simulink model "block_diagram_for_three_phase_vsi"  (R2014a)
settings: Solver=ode23t  StartTime=0.0  StopTime=1  MaxStep=1e-6  RelTol=1e-3
values from neighbouring files (symbols this model uses):
  p11 = rem(m,360)    [code_for_single_phase_csi.m]    (also in code_for_single_phase_vsi.m; code_for_three_phase_csi.m; code_for_three_phase_vsi.m; code_for_vsi.m)
  p22 = rem(n,360)    [code_for_single_phase_csi.m]    (also in code_for_single_phase_vsi.m; code_for_three_phase_csi.m; code_for_three_phase_vsi.m; code_for_vsi.m)
  p33 = rem(o,360)    [code_for_single_phase_csi.m]    (also in code_for_single_phase_vsi.m; code_for_three_phase_csi.m; code_for_three_phase_vsi.m; code_for_vsi.m)
  p44 = rem(p,360)    [code_for_single_phase_csi.m]    (also in code_for_single_phase_vsi.m; code_for_three_phase_csi.m; code_for_three_phase_vsi.m; code_for_vsi.m)
  p55 = rem(q,360)    [code_for_single_phase_csi.m]    (also in code_for_single_phase_vsi.m; code_for_three_phase_csi.m; code_for_three_phase_vsi.m; code_for_vsi.m)
  p66 = rem(r,360)    [code_for_single_phase_csi.m]    (also in code_for_single_phase_vsi.m; code_for_three_phase_csi.m; code_for_three_phase_vsi.m; code_for_vsi.m)
  p77 = rem(s,360)    [code_for_single_phase_csi.m]    (also in code_for_single_phase_vsi.m; code_for_three_phase_csi.m; code_for_three_phase_vsi.m; code_for_vsi.m)
  p88 = rem(t,360)    [code_for_three_phase_vsi.m]    (also in code_for_vsi.m)
libraries: powerlib x16, powerlib_meascontrol x2
settings Model: Creator=singa  LastModifiedBy=singa

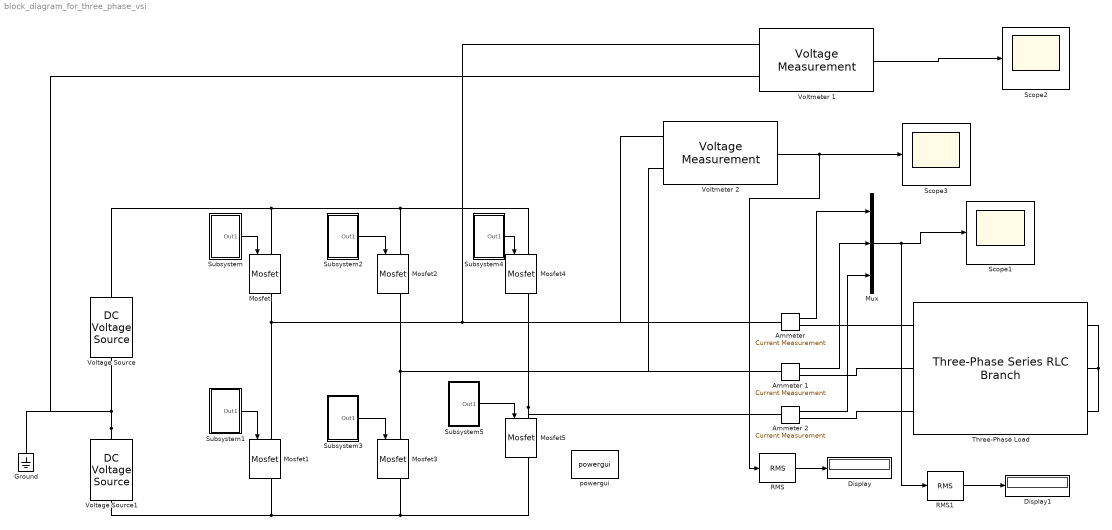
== system block_diagram_for_three_phase_vsi ==
  Ammeter : powerlib/Measurements/Current Measurement  PhasorSimulation=off  OutputType=Complex  PSBequivalent=0
  Ammeter 1 : powerlib/Measurements/Current Measurement  PhasorSimulation=off  OutputType=Complex  PSBequivalent=0
  Ammeter 2 : powerlib/Measurements/Current Measurement  PhasorSimulation=off  OutputType=Complex  PSBequivalent=0
  Display : Display
  Display1 : Display
  Ground : powerlib/Elements/Ground  LConnTagsString=a
  Mosfet{,1..5} (6 alike) : powerlib/Power Electronics/Mosfet  Ron=0.1  Lon=0  Rd=0.01  Vfd=0  IC=0  Rs=1e5  Cs=inf  Measurements=on
  Mux : Mux  Inputs=3
  RMS : powerlib_meascontrol/Measurements/RMS  TrueRMS=on  Freq=50  RMSInit=0  Ts=0
  RMS1 : powerlib_meascontrol/Measurements/RMS  TrueRMS=on  Freq=50  RMSInit=0  Ts=0
  Scope1 : Scope
      settings: YMin=-30  YMax=30  SampleInput=on  SampleTime=1e-6
  Scope2 : Scope
      settings: YMin=-200  YMax=200  SaveName=ScopeData2  SampleInput=on  SampleTime=1e-6
  Scope3 : Scope
      settings: TimeRange=1  YMin=-200  YMax=200  SaveName=ScopeData3  SampleInput=on  SampleTime=1e-6
  Subsystem : Subsystem
  Subsystem1 : Subsystem
  Subsystem2 : Subsystem
  Subsystem3 : Subsystem
  Subsystem4 : Subsystem
  Subsystem5 : Subsystem
  Three-Phase Load : powerlib/Elements/Three-Phase Series RLC Branch  LConnTagsString=A|B|C  RConnTagsString=A|B|C  BranchType=RL  Resistance=1  Inductance=0.01  Capacitance=1e-6  Measurements=None
  Voltage Source : powerlib/Electrical Sources/DC Voltage Source  Amplitude=50  Measurements=None
  Voltage Source1 : powerlib/Electrical Sources/DC Voltage Source  Amplitude=50  Measurements=None
  Voltmeter 1 : powerlib/Measurements/Voltage Measurement  PhasorSimulation=off  OutputType=Complex  PSBequivalent=0
  Voltmeter 2 : powerlib/Measurements/Voltage Measurement  PhasorSimulation=off  OutputType=Complex  PSBequivalent=0
  powergui : powerlib/powergui  Priority=1  SimulationMode=Continuous  SolverType=Tustin  SampleTime=50e-6  frequency=60  SPID=off  DisableSnubberDevices=off  DisableRonSwitches=off  DisableVfSwitches=off  SwTol=0  Interpol=off  DisplayEquations=off  Ts=0  methode=off  frequencyindice=0  Pbase=100e6  ErrMax=1e-4  Iterations=50  UnitsV=kV  UnitsW=MW  FunctionMessages=off  echomessages=off  HookPort=off  EnableUseOfTLC=off  x0status=blocks  RestoreLinks=warning  ResistiveCurrentMeasurement=off  Frange=[0:2:500]  Ylog=off  Xlog=on  ShowGrid=off  save=off  variable=ZData  structure=ScopeData1  ZoomFFT=off  StartTime=0.75  cycles=2  DisplayStyle=4  fundamental=50  FreqAxis=on  MaxFrequency=2500  frequencyindicesteady=1  RmsSteady=1  display=off
  wires:
  Ammeter/1 -> Mux/1
  Ammeter 1/1 -> Mux/2
  Ammeter 2/1 -> Mux/3
  Mux/1 -> RMS1/1, Scope1/1
  Voltmeter 1/1 -> Scope2/1
  Subsystem/1(Out1) -> Mosfet/1
  Subsystem1/1(Out1) -> Mosfet1/1
  Subsystem2/1(Out1) -> Mosfet2/1
  Subsystem3/1(Out1) -> Mosfet3/1
  Subsystem4/1(Out1) -> Mosfet4/1
  Subsystem5/1(Out1) -> Mosfet5/1
  Voltmeter 2/1 -> RMS/1, Scope3/1
  RMS/1 -> Display/1
  RMS1/1 -> Display1/1
  connections:
  Voltage Source1/RConn1 -- Voltmeter 1/LConn2 -- Ground/LConn1 -- Voltage Source/LConn1
  Mosfet/RConn1 -- Voltmeter 2/LConn1 -- Ammeter/LConn1 -- Voltmeter 1/LConn1 -- Mosfet1/LConn1
  Mosfet2/RConn1 -- Voltmeter 2/LConn2 -- Ammeter 1/LConn1 -- Mosfet3/LConn1
  Mosfet4/RConn1 -- Ammeter 2/LConn1 -- Mosfet5/LConn1
  Mosfet/LConn1 -- Mosfet4/LConn1 -- Mosfet2/LConn1 -- Voltage Source/RConn1
  Mosfet1/RConn1 -- Voltage Source1/LConn1 -- Mosfet3/RConn1 -- Mosfet5/RConn1
  Three-Phase Load/RConn1 -- Three-Phase Load/RConn3 -- Three-Phase Load/RConn2
  Ammeter/RConn1 -- Three-Phase Load/LConn1
  Ammeter 1/RConn1 -- Three-Phase Load/LConn2
  Ammeter 2/RConn1 -- Three-Phase Load/LConn3

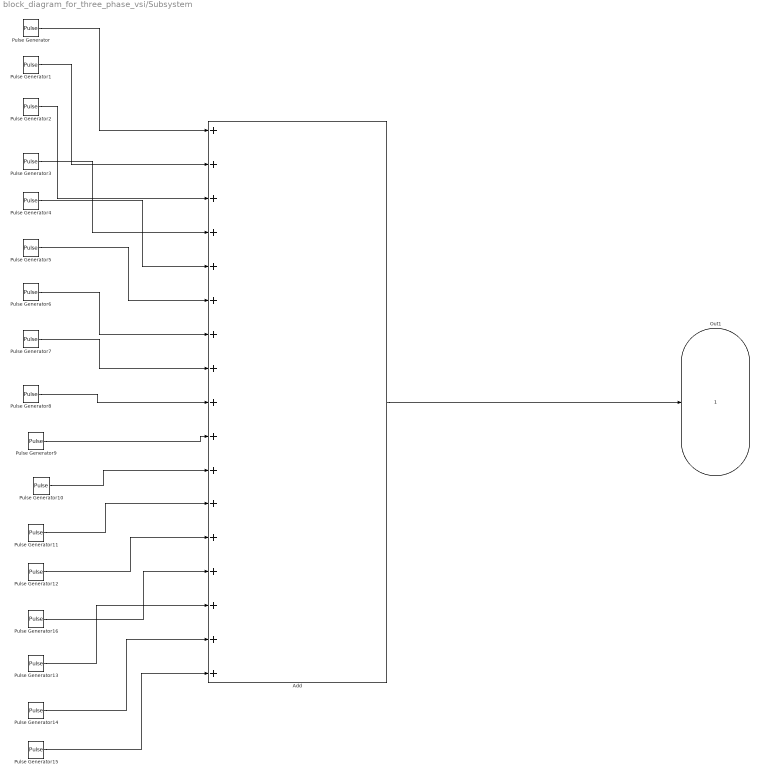
== system block_diagram_for_three_phase_vsi/Subsystem ==
  Add : Sum  Inputs=+++++++++++++++++
  Pulse Generator : DiscretePulseGenerator  PulseType=Time based  Period=0.02  PulseWidth=(p11/360)*100
  Pulse Generator1 : DiscretePulseGenerator  PulseType=Time based  Period=0.02  PulseWidth=(p33-p22)/360*100  PhaseDelay=p22/360*0.02
  Pulse Generator10 : DiscretePulseGenerator  PulseType=Time based  Period=0.02  PulseWidth=(p44-p33)/360*100  PhaseDelay=0.01+p33/360*0.02
  Pulse Generator11 : DiscretePulseGenerator  PulseType=Time based  Period=0.02  PulseWidth=(p66-p55)/360*100  PhaseDelay=0.01+p55/360*0.02
  Pulse Generator12 : DiscretePulseGenerator  PulseType=Time based  Period=0.02  PulseWidth=(p88-p77)/360*100  PhaseDelay=0.01+p77/360*0.02
  Pulse Generator13 : DiscretePulseGenerator  PulseType=Time based  Period=0.02  PulseWidth=(p66-p55)/360*100  PhaseDelay=0.01+(180-p66)/360*0.02
  Pulse Generator14 : DiscretePulseGenerator  PulseType=Time based  Period=0.02  PulseWidth=(p44-p33)/360*100  PhaseDelay=0.01+(180-p44)/360*0.02
  Pulse Generator15 : DiscretePulseGenerator  PulseType=Time based  Period=0.02  PulseWidth=(p22-p11)/360*100  PhaseDelay=0.01+(180-p22)/360*0.02
  Pulse Generator16 : DiscretePulseGenerator  PulseType=Time based  Period=0.02  PulseWidth=(p88-p77)/360*100  PhaseDelay=0.01+(180-p88)/360*0.02
  Pulse Generator2 : DiscretePulseGenerator  PulseType=Time based  Period=0.02  PulseWidth=(p55-p44)/360*100  PhaseDelay=p44/360*0.02
  Pulse Generator3 : DiscretePulseGenerator  PulseType=Time based  Period=0.02  PulseWidth=(p77-p66)/360*100  PhaseDelay=p66/360*0.02
  Pulse Generator4 : DiscretePulseGenerator  PulseType=Time based  Period=0.02  PulseWidth=(90-p88)/180*100  PhaseDelay=p88/360*0.02
  Pulse Generator5 : DiscretePulseGenerator  PulseType=Time based  Period=0.02  PulseWidth=(p77-p66)/360*100  PhaseDelay=(180-p77)/360*0.02
  Pulse Generator6 : DiscretePulseGenerator  PulseType=Time based  Period=0.02  PulseWidth=(p55-p44)/360*100  PhaseDelay=(180-p55)/360*0.02
  Pulse Generator7 : DiscretePulseGenerator  PulseType=Time based  Period=0.02  PulseWidth=(p33-p22)/360*100  PhaseDelay=(180-p33)/360*0.02
  Pulse Generator8 : DiscretePulseGenerator  PulseType=Time based  Period=0.02  PulseWidth=(p11/360)*100  PhaseDelay=(180-p11)/360*0.02
  Pulse Generator9 : DiscretePulseGenerator  PulseType=Time based  Period=0.02  PulseWidth=(p22-p11)/360*100  PhaseDelay=0.01+p11/360*0.02
  Out1 : Outport
  wires:
  Pulse Generator4/1 -> Add/5
  Pulse Generator15/1 -> Add/17
  Pulse Generator6/1 -> Add/7
  Pulse Generator7/1 -> Add/8
  Pulse Generator16/1 -> Add/14
  Pulse Generator5/1 -> Add/6
  Pulse Generator9/1 -> Add/10
  Pulse Generator2/1 -> Add/3
  Pulse Generator12/1 -> Add/13
  Pulse Generator10/1 -> Add/11
  Pulse Generator11/1 -> Add/12
  Pulse Generator3/1 -> Add/4
  Pulse Generator1/1 -> Add/2
  Pulse Generator/1 -> Add/1
  Pulse Generator13/1 -> Add/15
  Pulse Generator14/1 -> Add/16
  Pulse Generator8/1 -> Add/9
  Add/1 -> Out1/1

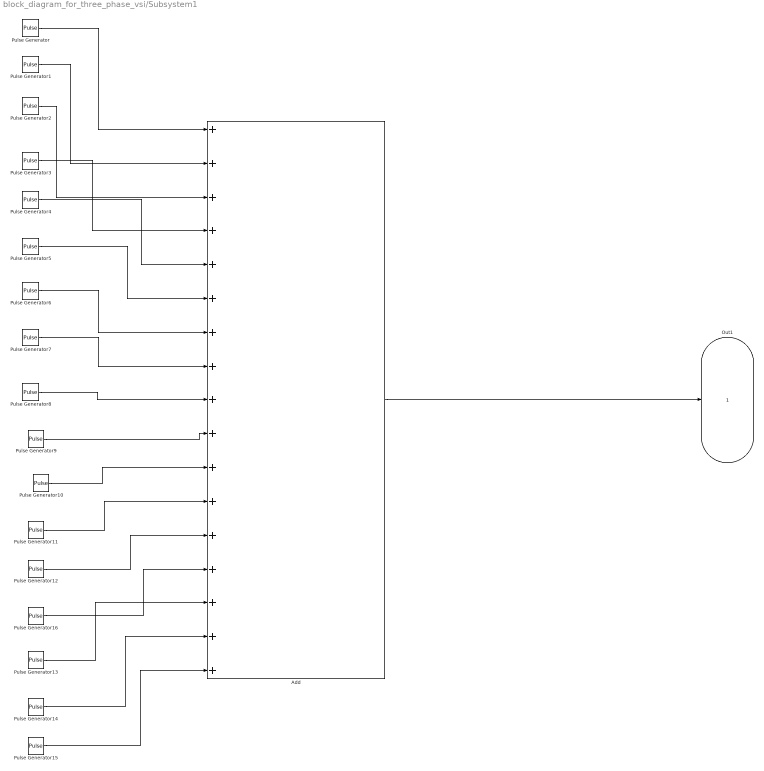
== system block_diagram_for_three_phase_vsi/Subsystem1 ==
  Add : Sum  Inputs=+++++++++++++++++
  Pulse Generator : DiscretePulseGenerator  PulseType=Time based  Period=0.02  PulseWidth=(p11/360)*100  PhaseDelay=0.01
  Pulse Generator1 : DiscretePulseGenerator  PulseType=Time based  Period=0.02  PulseWidth=(p33-p22)/360*100  PhaseDelay=p22/360*0.02+0.01
  Pulse Generator10 : DiscretePulseGenerator  PulseType=Time based  Period=0.02  PulseWidth=(p44-p33)/360*100  PhaseDelay=0.01+p33/360*0.02+0.01
  Pulse Generator11 : DiscretePulseGenerator  PulseType=Time based  Period=0.02  PulseWidth=(p66-p55)/360*100  PhaseDelay=0.01+p55/360*0.02+0.01
  Pulse Generator12 : DiscretePulseGenerator  PulseType=Time based  Period=0.02  PulseWidth=(p88-p77)/360*100  PhaseDelay=0.01+p77/360*0.02+0.01
  Pulse Generator13 : DiscretePulseGenerator  PulseType=Time based  Period=0.02  PulseWidth=(p66-p55)/360*100  PhaseDelay=0.01+(180-p66)/360*0.02+0.01
  Pulse Generator14 : DiscretePulseGenerator  PulseType=Time based  Period=0.02  PulseWidth=(p44-p33)/360*100  PhaseDelay=0.01+(180-p44)/360*0.02+0.01
  Pulse Generator15 : DiscretePulseGenerator  PulseType=Time based  Period=0.02  PulseWidth=(p22-p11)/360*100  PhaseDelay=0.01+(180-p22)/360*0.02+0.01
  Pulse Generator16 : DiscretePulseGenerator  PulseType=Time based  Period=0.02  PulseWidth=(p88-p77)/360*100  PhaseDelay=0.01+(180-p88)/360*0.02+0.01
  Pulse Generator2 : DiscretePulseGenerator  PulseType=Time based  Period=0.02  PulseWidth=(p55-p44)/360*100  PhaseDelay=p44/360*0.02+0.01
  Pulse Generator3 : DiscretePulseGenerator  PulseType=Time based  Period=0.02  PulseWidth=(p77-p66)/360*100  PhaseDelay=p66/360*0.02+0.01
  Pulse Generator4 : DiscretePulseGenerator  PulseType=Time based  Period=0.02  PulseWidth=(90-p88)/180*100  PhaseDelay=p88/360*0.02+0.01
  Pulse Generator5 : DiscretePulseGenerator  PulseType=Time based  Period=0.02  PulseWidth=(p77-p66)/360*100  PhaseDelay=(180-p77)/360*0.02+0.01
  Pulse Generator6 : DiscretePulseGenerator  PulseType=Time based  Period=0.02  PulseWidth=(p55-p44)/360*100  PhaseDelay=(180-p55)/360*0.02+0.01
  Pulse Generator7 : DiscretePulseGenerator  PulseType=Time based  Period=0.02  PulseWidth=(p33-p22)/360*100  PhaseDelay=(180-p33)/360*0.02+0.01
  Pulse Generator8 : DiscretePulseGenerator  PulseType=Time based  Period=0.02  PulseWidth=(p11/360)*100  PhaseDelay=(180-p11)/360*0.02+0.01
  Pulse Generator9 : DiscretePulseGenerator  PulseType=Time based  Period=0.02  PulseWidth=(p22-p11)/360*100  PhaseDelay=0.01+p11/360*0.02+0.01
  Out1 : Outport
  wires:
  Add/1 -> Out1/1
  Pulse Generator4/1 -> Add/5
  Pulse Generator15/1 -> Add/17
  Pulse Generator6/1 -> Add/7
  Pulse Generator7/1 -> Add/8
  Pulse Generator16/1 -> Add/14
  Pulse Generator5/1 -> Add/6
  Pulse Generator9/1 -> Add/10
  Pulse Generator2/1 -> Add/3
  Pulse Generator12/1 -> Add/13
  Pulse Generator10/1 -> Add/11
  Pulse Generator11/1 -> Add/12
  Pulse Generator3/1 -> Add/4
  Pulse Generator1/1 -> Add/2
  Pulse Generator/1 -> Add/1
  Pulse Generator13/1 -> Add/15
  Pulse Generator14/1 -> Add/16
  Pulse Generator8/1 -> Add/9

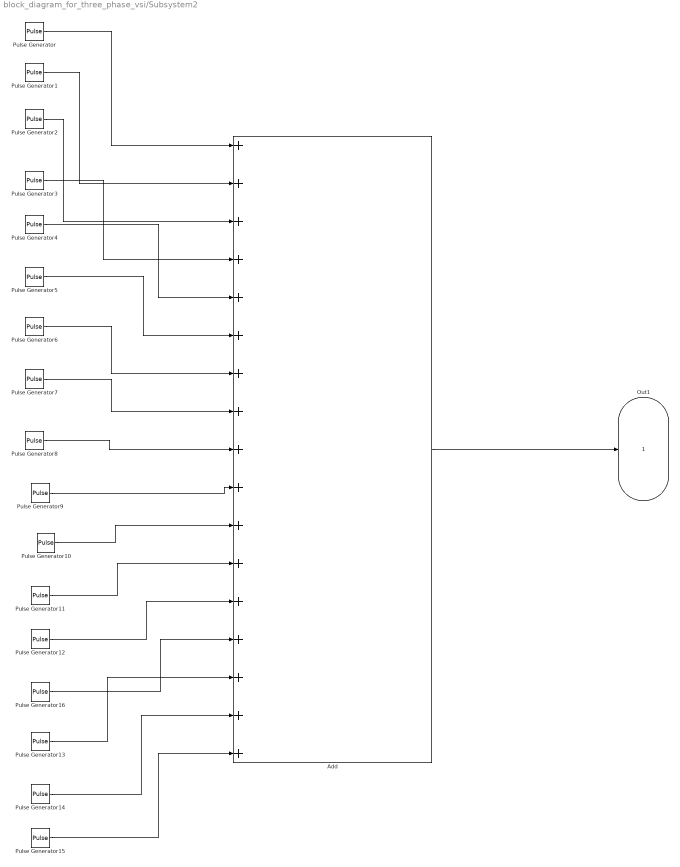
== system block_diagram_for_three_phase_vsi/Subsystem2 ==
  Add : Sum  Inputs=+++++++++++++++++
  Pulse Generator : DiscretePulseGenerator  PulseType=Time based  Period=0.02  PulseWidth=(p11/360)*100  PhaseDelay=0.02/3
  Pulse Generator1 : DiscretePulseGenerator  PulseType=Time based  Period=0.02  PulseWidth=(p33-p22)/360*100  PhaseDelay=p22/360*0.02+0.02/3
  Pulse Generator10 : DiscretePulseGenerator  PulseType=Time based  Period=0.02  PulseWidth=(p44-p33)/360*100  PhaseDelay=0.01+p33/360*0.02+0.02/3
  Pulse Generator11 : DiscretePulseGenerator  PulseType=Time based  Period=0.02  PulseWidth=(p66-p55)/360*100  PhaseDelay=0.01+p55/360*0.02+0.02/3
  Pulse Generator12 : DiscretePulseGenerator  PulseType=Time based  Period=0.02  PulseWidth=(p88-p77)/360*100  PhaseDelay=0.01+p77/360*0.02+0.02/3
  Pulse Generator13 : DiscretePulseGenerator  PulseType=Time based  Period=0.02  PulseWidth=(p66-p55)/360*100  PhaseDelay=0.01+(180-p66)/360*0.02+0.02/3
  Pulse Generator14 : DiscretePulseGenerator  PulseType=Time based  Period=0.02  PulseWidth=(p44-p33)/360*100  PhaseDelay=0.01+(180-p44)/360*0.02+0.02/3
  Pulse Generator15 : DiscretePulseGenerator  PulseType=Time based  Period=0.02  PulseWidth=(p22-p11)/360*100  PhaseDelay=0.01+(180-p22)/360*0.02+0.02/3
  Pulse Generator16 : DiscretePulseGenerator  PulseType=Time based  Period=0.02  PulseWidth=(p88-p77)/360*100  PhaseDelay=0.01+(180-p88)/360*0.02+0.02/3
  Pulse Generator2 : DiscretePulseGenerator  PulseType=Time based  Period=0.02  PulseWidth=(p55-p44)/360*100  PhaseDelay=p44/360*0.02+0.02/3
  Pulse Generator3 : DiscretePulseGenerator  PulseType=Time based  Period=0.02  PulseWidth=(p77-p66)/360*100  PhaseDelay=p66/360*0.02+0.02/3
  Pulse Generator4 : DiscretePulseGenerator  PulseType=Time based  Period=0.02  PulseWidth=(90-p88)/180*100  PhaseDelay=p88/360*0.02+0.02/3
  Pulse Generator5 : DiscretePulseGenerator  PulseType=Time based  Period=0.02  PulseWidth=(p77-p66)/360*100  PhaseDelay=(180-p77)/360*0.02+0.02/3
  Pulse Generator6 : DiscretePulseGenerator  PulseType=Time based  Period=0.02  PulseWidth=(p55-p44)/360*100  PhaseDelay=(180-p55)/360*0.02+0.02/3
  Pulse Generator7 : DiscretePulseGenerator  PulseType=Time based  Period=0.02  PulseWidth=(p33-p22)/360*100  PhaseDelay=(180-p33)/360*0.02+0.02/3
  Pulse Generator8 : DiscretePulseGenerator  PulseType=Time based  Period=0.02  PulseWidth=(p11/360)*100  PhaseDelay=(180-p11)/360*0.02+0.02/3
  Pulse Generator9 : DiscretePulseGenerator  PulseType=Time based  Period=0.02  PulseWidth=(p22-p11)/360*100  PhaseDelay=0.01+p11/360*0.02+0.02/3
  Out1 : Outport
  wires:
  Add/1 -> Out1/1
  Pulse Generator4/1 -> Add/5
  Pulse Generator15/1 -> Add/17
  Pulse Generator6/1 -> Add/7
  Pulse Generator7/1 -> Add/8
  Pulse Generator16/1 -> Add/14
  Pulse Generator5/1 -> Add/6
  Pulse Generator9/1 -> Add/10
  Pulse Generator2/1 -> Add/3
  Pulse Generator12/1 -> Add/13
  Pulse Generator10/1 -> Add/11
  Pulse Generator11/1 -> Add/12
  Pulse Generator3/1 -> Add/4
  Pulse Generator1/1 -> Add/2
  Pulse Generator/1 -> Add/1
  Pulse Generator13/1 -> Add/15
  Pulse Generator14/1 -> Add/16
  Pulse Generator8/1 -> Add/9

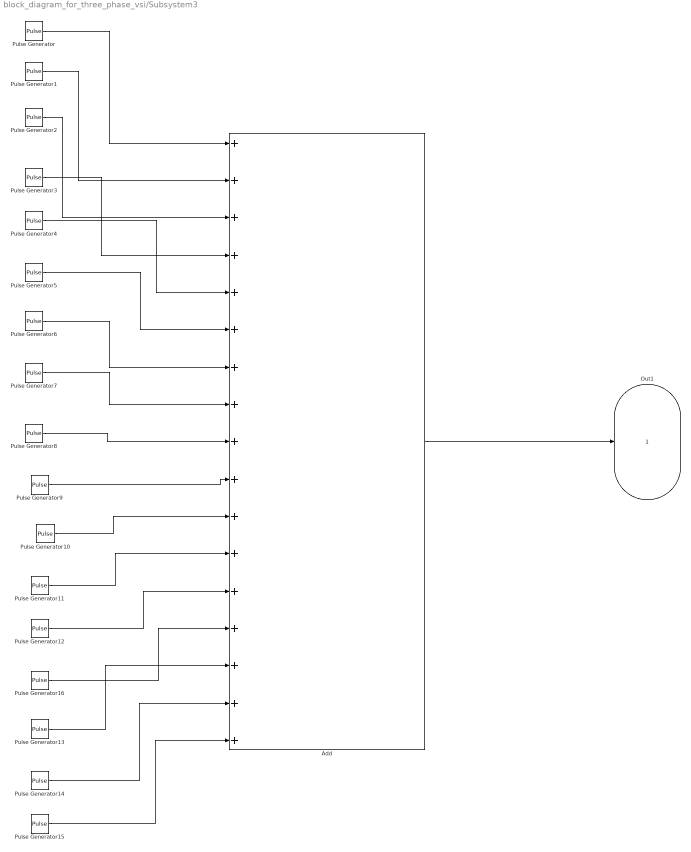
== system block_diagram_for_three_phase_vsi/Subsystem3 ==
  Add : Sum  Inputs=+++++++++++++++++
  Pulse Generator : DiscretePulseGenerator  PulseType=Time based  Period=0.02  PulseWidth=(p11/360)*100  PhaseDelay=0.01+0.02/3
  Pulse Generator1 : DiscretePulseGenerator  PulseType=Time based  Period=0.02  PulseWidth=(p33-p22)/360*100  PhaseDelay=p22/360*0.02+0.01+0.02/3
  Pulse Generator10 : DiscretePulseGenerator  PulseType=Time based  Period=0.02  PulseWidth=(p44-p33)/360*100  PhaseDelay=0.01+p33/360*0.02+0.01+0.02/3
  Pulse Generator11 : DiscretePulseGenerator  PulseType=Time based  Period=0.02  PulseWidth=(p66-p55)/360*100  PhaseDelay=0.01+p55/360*0.02+0.01+0.02/3
  Pulse Generator12 : DiscretePulseGenerator  PulseType=Time based  Period=0.02  PulseWidth=(p88-p77)/360*100  PhaseDelay=0.01+p77/360*0.02+0.01+0.02/3
  Pulse Generator13 : DiscretePulseGenerator  PulseType=Time based  Period=0.02  PulseWidth=(p66-p55)/360*100  PhaseDelay=0.01+(180-p66)/360*0.02+0.01+0.02/3
  Pulse Generator14 : DiscretePulseGenerator  PulseType=Time based  Period=0.02  PulseWidth=(p44-p33)/360*100  PhaseDelay=0.01+(180-p44)/360*0.02+0.01+0.02/3
  Pulse Generator15 : DiscretePulseGenerator  PulseType=Time based  Period=0.02  PulseWidth=(p22-p11)/360*100  PhaseDelay=0.01+(180-p22)/360*0.02+0.01+0.02/3
  Pulse Generator16 : DiscretePulseGenerator  PulseType=Time based  Period=0.02  PulseWidth=(p88-p77)/360*100  PhaseDelay=0.01+(180-p88)/360*0.02+0.01+0.02/3
  Pulse Generator2 : DiscretePulseGenerator  PulseType=Time based  Period=0.02  PulseWidth=(p55-p44)/360*100  PhaseDelay=p44/360*0.02+0.01+0.02/3
  Pulse Generator3 : DiscretePulseGenerator  PulseType=Time based  Period=0.02  PulseWidth=(p77-p66)/360*100  PhaseDelay=p66/360*0.02+0.01+0.02/3
  Pulse Generator4 : DiscretePulseGenerator  PulseType=Time based  Period=0.02  PulseWidth=(90-p88)/180*100  PhaseDelay=p88/360*0.02+0.01+0.02/3
  Pulse Generator5 : DiscretePulseGenerator  PulseType=Time based  Period=0.02  PulseWidth=(p77-p66)/360*100  PhaseDelay=(180-p77)/360*0.02+0.01+0.02/3
  Pulse Generator6 : DiscretePulseGenerator  PulseType=Time based  Period=0.02  PulseWidth=(p55-p44)/360*100  PhaseDelay=(180-p55)/360*0.02+0.01+0.02/3
  Pulse Generator7 : DiscretePulseGenerator  PulseType=Time based  Period=0.02  PulseWidth=(p33-p22)/360*100  PhaseDelay=(180-p33)/360*0.02+0.01+0.02/3
  Pulse Generator8 : DiscretePulseGenerator  PulseType=Time based  Period=0.02  PulseWidth=(p11/360)*100  PhaseDelay=(180-p11)/360*0.02+0.01+0.02/3
  Pulse Generator9 : DiscretePulseGenerator  PulseType=Time based  Period=0.02  PulseWidth=(p22-p11)/360*100  PhaseDelay=0.01+p11/360*0.02+0.01+0.02/3
  Out1 : Outport
  wires:
  Add/1 -> Out1/1
  Pulse Generator4/1 -> Add/5
  Pulse Generator15/1 -> Add/17
  Pulse Generator6/1 -> Add/7
  Pulse Generator7/1 -> Add/8
  Pulse Generator16/1 -> Add/14
  Pulse Generator5/1 -> Add/6
  Pulse Generator9/1 -> Add/10
  Pulse Generator2/1 -> Add/3
  Pulse Generator12/1 -> Add/13
  Pulse Generator10/1 -> Add/11
  Pulse Generator11/1 -> Add/12
  Pulse Generator3/1 -> Add/4
  Pulse Generator1/1 -> Add/2
  Pulse Generator/1 -> Add/1
  Pulse Generator13/1 -> Add/15
  Pulse Generator14/1 -> Add/16
  Pulse Generator8/1 -> Add/9

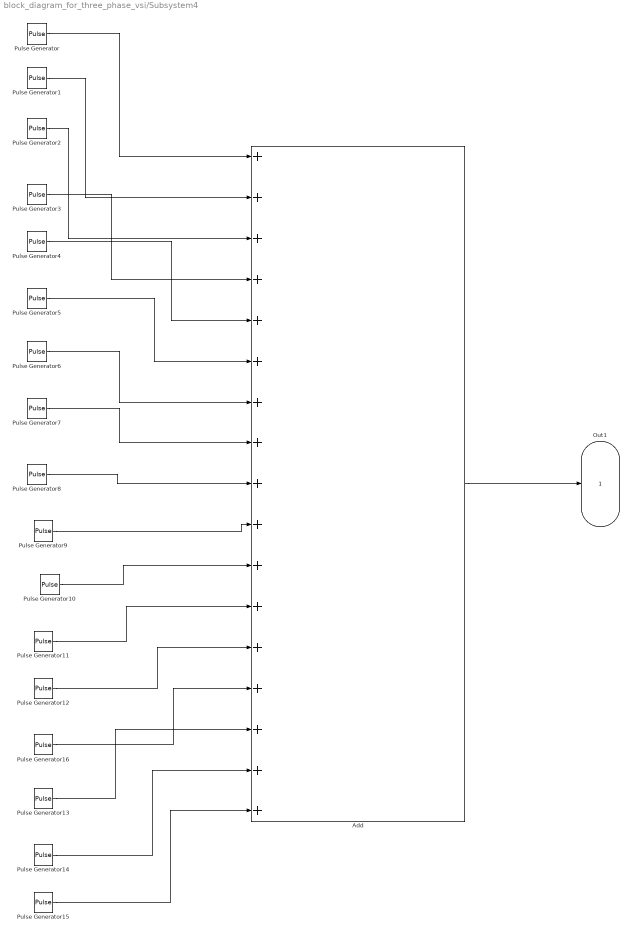
== system block_diagram_for_three_phase_vsi/Subsystem4 ==
  Add : Sum  Inputs=+++++++++++++++++
  Pulse Generator : DiscretePulseGenerator  PulseType=Time based  Period=0.02  PulseWidth=(p11/360)*100  PhaseDelay=0.04/3
  Pulse Generator1 : DiscretePulseGenerator  PulseType=Time based  Period=0.02  PulseWidth=(p33-p22)/360*100  PhaseDelay=p22/360*0.02+0.04/3
  Pulse Generator10 : DiscretePulseGenerator  PulseType=Time based  Period=0.02  PulseWidth=(p44-p33)/360*100  PhaseDelay=0.01+p33/360*0.02+0.04/3
  Pulse Generator11 : DiscretePulseGenerator  PulseType=Time based  Period=0.02  PulseWidth=(p66-p55)/360*100  PhaseDelay=0.01+p55/360*0.02+0.04/3
  Pulse Generator12 : DiscretePulseGenerator  PulseType=Time based  Period=0.02  PulseWidth=(p88-p77)/360*100  PhaseDelay=0.01+p77/360*0.02+0.04/3
  Pulse Generator13 : DiscretePulseGenerator  PulseType=Time based  Period=0.02  PulseWidth=(p66-p55)/360*100  PhaseDelay=0.01+(180-p66)/360*0.02+0.04/3
  Pulse Generator14 : DiscretePulseGenerator  PulseType=Time based  Period=0.02  PulseWidth=(p44-p33)/360*100  PhaseDelay=0.01+(180-p44)/360*0.02+0.04/3
  Pulse Generator15 : DiscretePulseGenerator  PulseType=Time based  Period=0.02  PulseWidth=(p22-p11)/360*100  PhaseDelay=0.01+(180-p22)/360*0.02+0.04/3
  Pulse Generator16 : DiscretePulseGenerator  PulseType=Time based  Period=0.02  PulseWidth=(p88-p77)/360*100  PhaseDelay=0.01+(180-p88)/360*0.02+0.04/3
  Pulse Generator2 : DiscretePulseGenerator  PulseType=Time based  Period=0.02  PulseWidth=(p55-p44)/360*100  PhaseDelay=p44/360*0.02+0.04/3
  Pulse Generator3 : DiscretePulseGenerator  PulseType=Time based  Period=0.02  PulseWidth=(p77-p66)/360*100  PhaseDelay=p66/360*0.02+0.04/3
  Pulse Generator4 : DiscretePulseGenerator  PulseType=Time based  Period=0.02  PulseWidth=(90-p88)/180*100  PhaseDelay=p88/360*0.02+0.04/3
  Pulse Generator5 : DiscretePulseGenerator  PulseType=Time based  Period=0.02  PulseWidth=(p77-p66)/360*100  PhaseDelay=(180-p77)/360*0.02+0.04/3
  Pulse Generator6 : DiscretePulseGenerator  PulseType=Time based  Period=0.02  PulseWidth=(p55-p44)/360*100  PhaseDelay=(180-p55)/360*0.02+0.04/3
  Pulse Generator7 : DiscretePulseGenerator  PulseType=Time based  Period=0.02  PulseWidth=(p33-p22)/360*100  PhaseDelay=(180-p33)/360*0.02+0.04/3
  Pulse Generator8 : DiscretePulseGenerator  PulseType=Time based  Period=0.02  PulseWidth=(p11/360)*100  PhaseDelay=(180-p11)/360*0.02+0.04/3
  Pulse Generator9 : DiscretePulseGenerator  PulseType=Time based  Period=0.02  PulseWidth=(p22-p11)/360*100  PhaseDelay=0.01+p11/360*0.02+0.04/3
  Out1 : Outport
  wires:
  Add/1 -> Out1/1
  Pulse Generator4/1 -> Add/5
  Pulse Generator15/1 -> Add/17
  Pulse Generator6/1 -> Add/7
  Pulse Generator7/1 -> Add/8
  Pulse Generator16/1 -> Add/14
  Pulse Generator5/1 -> Add/6
  Pulse Generator9/1 -> Add/10
  Pulse Generator2/1 -> Add/3
  Pulse Generator12/1 -> Add/13
  Pulse Generator10/1 -> Add/11
  Pulse Generator11/1 -> Add/12
  Pulse Generator3/1 -> Add/4
  Pulse Generator1/1 -> Add/2
  Pulse Generator/1 -> Add/1
  Pulse Generator13/1 -> Add/15
  Pulse Generator14/1 -> Add/16
  Pulse Generator8/1 -> Add/9

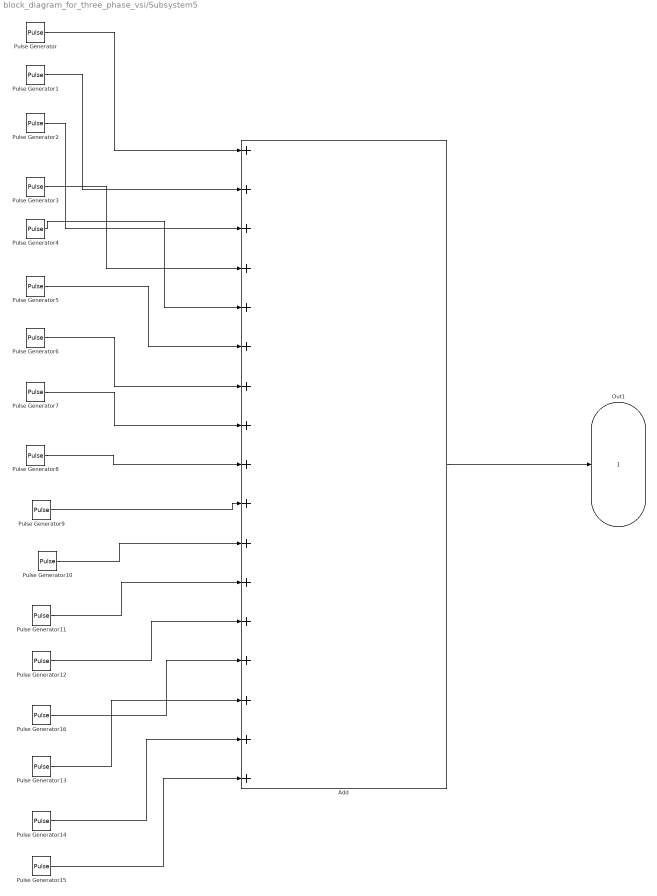
== system block_diagram_for_three_phase_vsi/Subsystem5 ==
  Add : Sum  Inputs=+++++++++++++++++
  Pulse Generator : DiscretePulseGenerator  PulseType=Time based  Period=0.02  PulseWidth=(p11/360)*100  PhaseDelay=0.01+0.04/3
  Pulse Generator1 : DiscretePulseGenerator  PulseType=Time based  Period=0.02  PulseWidth=(p33-p22)/360*100  PhaseDelay=p22/360*0.02+0.01+0.04/3
  Pulse Generator10 : DiscretePulseGenerator  PulseType=Time based  Period=0.02  PulseWidth=(p44-p33)/360*100  PhaseDelay=0.01+p33/360*0.02+0.01+0.04/3
  Pulse Generator11 : DiscretePulseGenerator  PulseType=Time based  Period=0.02  PulseWidth=(p66-p55)/360*100  PhaseDelay=0.01+p55/360*0.02+0.01+0.04/3
  Pulse Generator12 : DiscretePulseGenerator  PulseType=Time based  Period=0.02  PulseWidth=(p88-p77)/360*100  PhaseDelay=0.01+p77/360*0.02+0.01+0.04/3
  Pulse Generator13 : DiscretePulseGenerator  PulseType=Time based  Period=0.02  PulseWidth=(p66-p55)/360*100  PhaseDelay=0.01+(180-p66)/360*0.02+0.01+0.04/3
  Pulse Generator14 : DiscretePulseGenerator  PulseType=Time based  Period=0.02  PulseWidth=(p44-p33)/360*100  PhaseDelay=0.01+(180-p44)/360*0.02+0.01+0.04/3
  Pulse Generator15 : DiscretePulseGenerator  PulseType=Time based  Period=0.02  PulseWidth=(p22-p11)/360*100  PhaseDelay=0.01+(180-p22)/360*0.02+0.01+0.04/3
  Pulse Generator16 : DiscretePulseGenerator  PulseType=Time based  Period=0.02  PulseWidth=(p88-p77)/360*100  PhaseDelay=0.01+(180-p88)/360*0.02+0.01+0.04/3
  Pulse Generator2 : DiscretePulseGenerator  PulseType=Time based  Period=0.02  PulseWidth=(p55-p44)/360*100  PhaseDelay=p44/360*0.02+0.01+0.04/3
  Pulse Generator3 : DiscretePulseGenerator  PulseType=Time based  Period=0.02  PulseWidth=(p77-p66)/360*100  PhaseDelay=p66/360*0.02+0.01+0.04/3
  Pulse Generator4 : DiscretePulseGenerator  PulseType=Time based  Period=0.02  PulseWidth=(90-p88)/180*100  PhaseDelay=p88/360*0.02+0.01+0.04/3
  Pulse Generator5 : DiscretePulseGenerator  PulseType=Time based  Period=0.02  PulseWidth=(p77-p66)/360*100  PhaseDelay=(180-p77)/360*0.02+0.01+0.04/3
  Pulse Generator6 : DiscretePulseGenerator  PulseType=Time based  Period=0.02  PulseWidth=(p55-p44)/360*100  PhaseDelay=(180-p55)/360*0.02+0.01+0.04/3
  Pulse Generator7 : DiscretePulseGenerator  PulseType=Time based  Period=0.02  PulseWidth=(p33-p22)/360*100  PhaseDelay=(180-p33)/360*0.02+0.01+0.04/3
  Pulse Generator8 : DiscretePulseGenerator  PulseType=Time based  Period=0.02  PulseWidth=(p11/360)*100  PhaseDelay=(180-p11)/360*0.02+0.01+0.04/3
  Pulse Generator9 : DiscretePulseGenerator  PulseType=Time based  Period=0.02  PulseWidth=(p22-p11)/360*100  PhaseDelay=0.01+p11/360*0.02+0.01+0.04/3
  Out1 : Outport
  wires:
  Add/1 -> Out1/1
  Pulse Generator4/1 -> Add/5
  Pulse Generator15/1 -> Add/17
  Pulse Generator6/1 -> Add/7
  Pulse Generator7/1 -> Add/8
  Pulse Generator16/1 -> Add/14
  Pulse Generator5/1 -> Add/6
  Pulse Generator9/1 -> Add/10
  Pulse Generator2/1 -> Add/3
  Pulse Generator12/1 -> Add/13
  Pulse Generator10/1 -> Add/11
  Pulse Generator11/1 -> Add/12
  Pulse Generator3/1 -> Add/4
  Pulse Generator1/1 -> Add/2
  Pulse Generator/1 -> Add/1
  Pulse Generator13/1 -> Add/15
  Pulse Generator14/1 -> Add/16
  Pulse Generator8/1 -> Add/9
